simulink model "onecart"  (Simulink 6.0)
settings: Solver=ode23  SolverMode=SingleTasking  StartTime=0  StopTime=10000  MaxStep=0.1  RelTol=1e-3  AbsTol=1e-6
PreLoadFcn:
  | zeta=0.2;wn=1;
settings Model: Creator=The MathWorks Inc.  LastModifiedBy=batserve  ExtModeAutoUpdateStatusClock=off
settings DataIOCC: ExternalInput=[]  InitialState=[]  LimitDataPoints=off  SaveOutput=off  SaveTime=off
settings OptimizationCC: BooleanDataType=off
settings DebuggingCC: CheckExecutionContextPreStartOutputMsg=on  CheckExecutionContextRuntimeOutputMsg=on  SolverPrmCheckMsg=none
settings HardwareCC: TargetUnknown=on

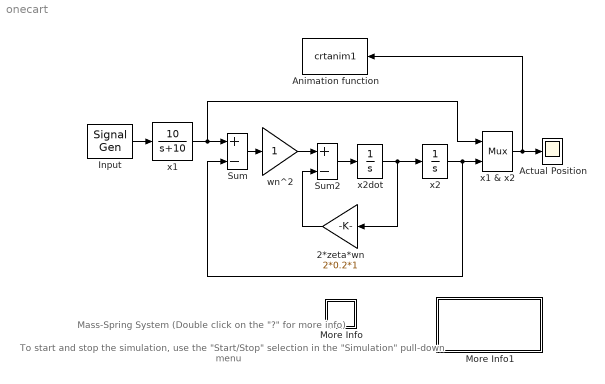
== system onecart ==
  note: Mass-Spring System
      | (Double click on the "?" for more info)
  note: To start and stop the simulation, use the "Start/Stop"
      | selection in the "Simulation" pull-down menu
  2*zeta*wn : Gain  Orientation=left  Gain=2*0.2*1  SaturateOnIntegerOverflow=on
  Actual Position : Scope
      settings: TickLabels=on  TimeRange=40.000000  DataFormat=Array
  Animation function : S-Function  Orientation=left  FunctionName=crtanim1  Parameters=.1
      settings: DeleteFcn=if ~isempty(findobj('type','figure','name','onecart Animation'));close('onecart Animation'); end;
  Input : SignalGenerator  WaveForm=square  Frequency=0.300000  Units=rad/sec
  More Info : Subsystem  PropExecContextAcrossSSBoundary=on
      mask Display: disp('?')
  More Info1 : Subsystem  PropExecContextAcrossSSBoundary=on
      settings: OpenFcn=simcad(bdroot);
      mask Display: disp('Double click\nhere for\nSimulink Help')
  Sum : Sum  Inputs=+-  SaturateOnIntegerOverflow=on  InputSameDT=on
  Sum2 : Sum  Inputs=+-  SaturateOnIntegerOverflow=on  InputSameDT=on
  wn^2 : Gain  SaturateOnIntegerOverflow=on
  x1 : TransferFcn  Numerator=10  Denominator=[1 10]
  x1 & x2 : Mux  Inputs=2
  x2 : Integrator
  x2dot : Integrator
  wires:
  Sum2/1 -> x2dot/1
  2*zeta*wn/1 -> Sum2/2
  wn^2/1 -> Sum2/1
  Sum/1 -> wn^2/1
  x2dot/1 -> x2/1, 2*zeta*wn/1
  x2/1 -> x1 & x2/2, Sum/2
  Input/1 -> x1/1
  x1 & x2/1 -> Animation function/1, Actual Position/1
  x1/1 -> Sum/1, x1 & x2/1

== system onecart/More Info ==
  note: Try experimenting with different initial conditions and
      | different settings for the forcing function.
  note: Associated with the demo is an animation function that
      | will automatically open a figure window and display to it.
  note: This system models a simple spring-mass-damper
      | system with a periodically varying forcing function.

== system onecart/More Info1 ==
  note: This system models a double pendulum system where
      | the rest state has both pendulums hanging vertically.
  note: Associated with the demo is an animation function that
      | will automatically open a figure window and display to it.
  note: Try experimenting with different initial conditions for
      | alpha and gamma to see the unusal coupling effects.
